simulink model "Simulasi_3DOFLengkap"  (R2024b)
settings: Solver=VariableStepAuto  StartTime=0.0  StopTime=500  FixedStep=au  RelTol=1e-10
values from neighbouring files (symbols this model uses):
  controller = 3    [Run_ILOS_PIDFUZZY.m]    (also in Run_ILOS_PIDMRAC.m; Run_PLOS_PID.m; Run_PLOS_PIDFUZZY.m = 2)
  gamma = 0.01    [Run_ILOS_PIDFUZZY.m]    (also in Run_ILOS_PIDMRAC.m; Run_PLOS_PID.m; Run_PLOS_PIDFUZZY.m)
  Gpi = [2 0.1]    [Run_ILOS_PIDFUZZY.m]    (also in Run_ILOS_PIDMRAC.m; Run_PLOS_PID.m; Run_PLOS_PIDFUZZY.m)
  guidance = 2    [Run_ILOS_PIDFUZZY.m]    (also in Run_ILOS_PIDMRAC.m; Run_PLOS_PID.m = 1; Run_PLOS_PIDFUZZY.m = 1)
  IzMinNrd = Iden(3)    [get_B.m]
  m = 11.8    [get_B.m]
  x_8 = [x_ling(1:50) x_ling(1:50)+40 x_ling(51:100)+40 x_ling(51:100)]    [Run_ILOS_PIDFUZZY.m]    (also in Run_ILOS_PIDMRAC.m; Run_PLOS_PID.m; Run_PLOS_PIDFUZZY.m)
  x_8e = [x_elips(1:50) x_elips(1:50)+60 x_elips(51:100)+60 x_elips(51:100)]    [Run_ILOS_PIDFUZZY.m]    (also in Run_ILOS_PIDMRAC.m; Run_PLOS_PID.m; Run_PLOS_PIDFUZZY.m)
  x_custom = [0 3 6 9 12 15 18 21 24 27 30 33 36 33 30 27 24 21 18 15 12 9 6 3 0]    [Run_ILOS_PIDFUZZY.m]    (also in Run_ILOS_PIDMRAC.m = [1 2 3 4 5 6]; Run_PLOS_PID.m; Run_PLOS_PIDFUZZY.m)
  x_elips = abs(x_elips)    [Run_ILOS_PIDFUZZY.m]    (also in Run_ILOS_PIDMRAC.m; Run_PLOS_PID.m; Run_PLOS_PIDFUZZY.m)
  x_ling = abs(x_ling)    [Run_ILOS_PIDFUZZY.m]    (also in Run_ILOS_PIDMRAC.m; Run_PLOS_PID.m; Run_PLOS_PIDFUZZY.m)
  x_s = [0 30 75 100]    [Run_ILOS_PIDMRAC.m]
  Xud = Iden(1)    [get_B.m]
  y_8 = [y_ling y_ling]    [Run_ILOS_PIDFUZZY.m]    (also in Run_ILOS_PIDMRAC.m; Run_PLOS_PID.m; Run_PLOS_PIDFUZZY.m)
  y_8e = [y_elips y_elips]    [Run_ILOS_PIDFUZZY.m]    (also in Run_ILOS_PIDMRAC.m; Run_PLOS_PID.m; Run_PLOS_PIDFUZZY.m)
  y_custom = [0 5 8 12 15 17 18 17 15 12 8 5 0 -5 -8 -12 -15 -17 -18 -17 -15 -12 -8 -5 0]    [Run_ILOS_PIDFUZZY.m]    (also in Run_ILOS_PIDMRAC.m = [10 10 10 10 10 10]; Run_PLOS_PID.m; Run_PLOS_PIDFUZZY.m)
  y_elips = 20 * sin(theta)    [Run_ILOS_PIDFUZZY.m]    (also in Run_ILOS_PIDMRAC.m; Run_PLOS_PID.m; Run_PLOS_PIDFUZZY.m)
  y_ling = radius * sin(theta)    [Run_ILOS_PIDFUZZY.m]    (also in Run_ILOS_PIDMRAC.m; Run_PLOS_PID.m; Run_PLOS_PIDFUZZY.m)
  y_s = [0 0 30 30]    [Run_ILOS_PIDMRAC.m]
undefined symbols (not defined in the file or in its folder): dr2, dr3, du2, du3, dv2, dv3, magnitude, Nr, Xu, Yv, Yvd
libraries: fuzblock x2, simulink x2, mssSimulink x1
(part 2 of 2)

== matlab function Simulasi_3DOFLengkap/USV 3 DOF ==
  data: V input; percepatan output size=3; T input; Te input; Yaw input; earth_d output size=3
function [percepatan,earth_d] = usv(V,T,Te,Yaw)

%vektor kecepatan searah sumbu x, y dan yaw
u=V(1);
v=V(2);
r=V(3);
u1 = u;
u2 = v;
u3 = r;
u4 = T(1);
u5 = T(3);

m = 11.8;

% % Variasi 1
Iden = [-32.7388185239266
-77.4849209555474
-104.663996293173
-25.6298484047442
0
0
-42.6421975895626
0
0
0
0
3.18087425146835
0
0
0
0
0
];

% % Variasi 3
% Iden = [-29.6348962860344
% -40.9001863942293
% -17.6979213719311
% -44.3102231335245
% 16.7610566258634
% -3.25974680868943
% -12.2481062983937
% -187.525882383106
% 242.293583318529
% 0
% 0
% 26.3914216879752
% -83.6415289921659
% 103.872584510861
% -0.567968563116999
% -31.9512915471382
% -0.876330232902557];

% % Variasi 2
Iden = [-27.1220584470477
-43.7904830700290
-23.5148195284010
-39.2219706313961
8.59337817510428
0
-42.8929067396088
7.06183045964360
0
0
0
9.53076811810547
12.6830530595321
0
-0.672629410917379
-40.3837561391473
-1.37052826486388];

Xud = Iden(1);
Yvd = Iden(2);
IzMinNrd = Iden(3);
Xu = Iden(4);
du2 = Iden(5);
du3 = Iden(6);

Yv =  Iden(7);
dv2 = Iden(8);
dv3 =Iden(9);
Yrv = Iden(10);
Yvr = Iden(11);

Nr = Iden(12);
dr2 = Iden(13);
dr3 = Iden(14);
Nrv = Iden(15);
Nvr =Iden(16);
Nvv = Iden(17);


% du2 = 0;
% du3 = 0;
% dv2 = 0;
% dv3 =0;
% dr2 =0;
% dr3 = 0;
% % % Dengan Gangguan
Te1 = Te(1);
Te2 = Te(2);
Te3 = Te(3);

% %Tanpa Gangguan


earth_d=[cos(Yaw) -sin(Yaw) 0; sin(Yaw) cos(Yaw) 0; 0 0 1]*V;
u_dot = 1/(m-Xud)*((m-Yvd)*u2*u3 + Xu*u1 - du2*abs(u1)*u1 + du3*(abs(u1)^2)*u1 + u4 +Te1) ;
v_dot = 1/(m-Yvd)*(-(m-Xud)*u1*u3 + Yv*u2 + dv2*abs(u2)*u2 + dv3*(abs(u2)^2)*u2 + Yrv*abs(u3)*u2 + Yvr*abs(u2)*u3 + Te2) ;
r_dot = 1/(IzMinNrd)*((Yvd-Xud)*u2*u1 + Nr*u3 + dr2*abs(u3)*u3 + dr3*(abs(u3)^2)*u3 + Nrv*abs(u3)*u2 + Nvr*abs(u2)*u3 + Nvv*abs(u2)*u2 + u5 +Te3) ;

%Output 
percepatan=[u_dot,v_dot,r_dot]';

== matlab function Simulasi_3DOFLengkap/Backup Tidak Digunakan/3 DOF/MATLAB Function ==
  data: V input; eta_d output; Yaw input
function eta_d = eta(V,Yaw)

eta_d=[cos(Yaw) sin(Yaw) 0; -sin(Yaw) cos(Yaw) 0; 0 0 1]*V;

== matlab function Simulasi_3DOFLengkap/MATLAB Function ==
  settings: updateMethod=DISCRETE
  data: x input; y input
% function realTimePlot(x, y, waypointX, waypointY)
% %#codegen
% coder.extrinsic('figure', 'plot', 'hold', 'grid', 'xlabel', 'ylabel', ...
%     'title', 'set', 'drawnow', 'isempty', 'gcf', 'xlim', 'ylim', 'legend');
% 
% % Persistent variables
% persistent xData yData hPlot fig hWaypoint;
% 
% % Inisialisasi variabel pada iterasi pertama
% if isempty(fig)
%     fig = figure('Name', 'Real-Time Plot', 'NumberTitle', 'off');
%     hold on;
%     grid on;
%     xlabel('X');
%     ylabel('Y');
%     title('Real-Time Plot of X vs Y with Waypoints');
%     xData = [];
%     yData = [];
%     hPlot = plot(NaN, NaN, 'b.-', 'MarkerSize', 10); % Plot lintasan
%     hWaypoint = plot(waypointX, waypointY, 'r--', 'MarkerSize', 1, 'LineWidth', 1); % Plot waypoint
%     legend('USV Path', 'Waypoint');
% end
% 
% % Pastikan dimensi konsisten
% if isrow(x)
%     x = x'; % Pastikan x adalah vektor kolom
% end
% if isrow(y)
%     y = y'; % Pastikan y adalah vektor kolom
% end
% 
% % Tambahkan data baru
% if isempty(xData)
%     xData = x; % Inisialisasi xData jika kosong
%     yData = y; % Inisialisasi yData jika kosong
% else
%     xData = [xData; x]; % Tambahkan data baru sebagai baris baru
%     yData = [yData; y]; % Tambahkan data baru sebagai baris baru
% end
% 
% % Perbarui plot lintasan
% set(hPlot, 'XData', xData, 'YData', yData);
% 
% % Perbarui waypoint (jika berubah)
% set(hWaypoint, 'XData', waypointX, 'YData', waypointY);
% % 
% % % Atur batas sumbu secara otomatis jika perlu
% % xlim([min([xData; waypointX]) - 5, max([xData; waypointX]) + 5]);
% % ylim([min([yData; waypointY]) - 5, max([yData; waypointY]) + 5]);
% 
% % Perbarui jendela plot
% drawnow;
% 
% end

function realTimePlot(x, y)
%#codegen
% Fungsi untuk menampilkan plot real-time dari input x dan y
% Input:
%   x - Nilai input x (titik pada sumbu X)
%   y - Nilai input y (titik pada sumbu Y)

% Deklarasikan fungsi grafik sebagai extrinsic
coder.extrinsic('figure', 'plot', 'hold', 'grid', 'xlabel', 'ylabel', ...
    'title', 'set', 'drawnow', 'isempty', 'gcf', 'xlim', 'ylim');

% Persistent variables
persistent xData yData hPlot fig;

% Inisialisasi variabel pada iterasi pertama
if isempty(fig)
    fig = figure('Name', 'Real-Time Plot', 'NumberTitle', 'off');
    hold on;
    grid on;
    xlabel('X');
    ylabel('Y');
    title('Real-Time Plot of X vs Y');
    xData = [];
    yData = [];
    hPlot = plot(NaN, NaN, 'b.-', 'MarkerSize', 10); % Buat plot awal
end

% Tambahkan data baru
xData = [xData, x];
yData = [yData, y];

% Perbarui plot
set(hPlot, 'XData', xData, 'YData', yData);

% Atur batas sumbu secara otomatis jika perlu
xlim([min(xData) - 1, max(xData) + 1]);
ylim([min(yData) - 1, max(yData) + 1]);

% Perbarui jendela plot
drawnow;

end

== matlab function Simulasi_3DOFLengkap/Backup Tidak Digunakan/Konversi Sinyal 1 ==
  data: Throttle input; Tu output; Tv output; Rudder input; Tr output; Vx input
function [Tu,Tv,Tr] = CV(Throttle,Rudder,Vx)
Kthrust = 0.0201;
Tu= Kthrust*1097.6*(1-exp(-13*abs(Throttle)/100));
Tv=0;
Tr = 18*(6.75*(10^-3)).*1.*Vx.^2.*(Rudder/100);

== matlab function Simulasi_3DOFLengkap/Subsystem/ALOS Guidance ==
  settings: updateMethod=DISCRETE
  data: x input; psi_d output; y input; Delta input; gamma input; R_switch input; xdata input; ydata input; U input; K_f input; h input; x_e output; y_e output; Gpi input
function [psi_d,x_e,y_e]= fcn(x,y,Delta,gamma,R_switch,xdata,ydata,U,K_f,h,Gpi)

% waypoints
wpt.pos.x = xdata;
wpt.pos.y = ydata;

% ALOS guidance law
[psi_d,x_e,y_e] = ALOSpsi(x,y,Delta,gamma,h,R_switch,wpt,U,K_f,Gpi);

end
